simulink model "ex_modeling_signals"  (R2019b)
settings: Solver=VariableStepAuto  StartTime=0.0  StopTime=30  RelTol=1e-3
libraries: simulink x2
settings Model: Creator=The MathWorks, Inc.  LastModifiedBy=The MathWorks, Inc.
settings DataIOCC: ReturnWorkspaceOutputs=off
settings DebuggingCC: PregeneratedLibrarySubsystemCodeDiagnostic=none  ArithmeticOperatorsInVariantConditions=warning
settings SFSimCC: SimUseLocalCustomCode=off  CustomCodeUndefinedFunction=UseInterfaceOnly
settings RTWCC: RTWUseLocalCustomCode=off

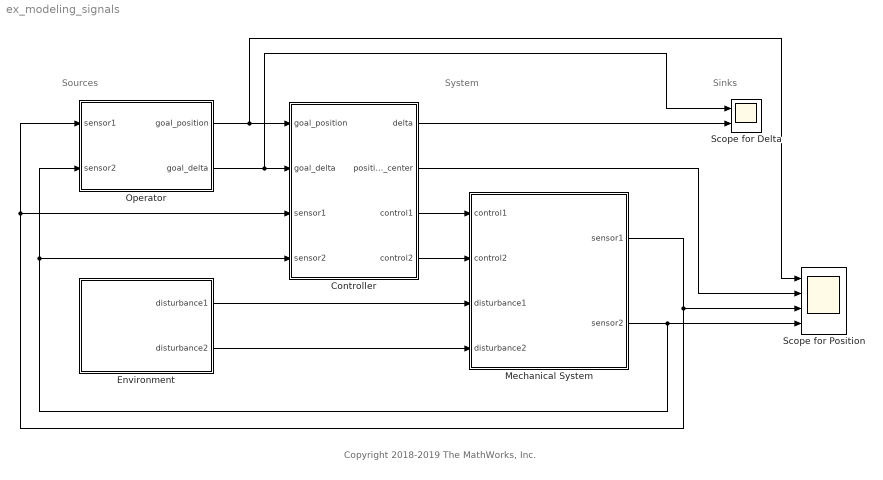
== system ex_modeling_signals ==
  note: System
  note: Sources
  note: Copyright 2018-2019 The MathWorks, Inc.
  note: Sinks
  Controller : Subsystem  TreatAsAtomicUnit=on
  Environment : Subsystem
  Mechanical System : Subsystem
  Operator : Subsystem
  Scope for Delta : Scope  NumInputPorts=2
  Scope for Position : Scope  NumInputPorts=4
  wires:
  Operator/1(goal_position) -> Controller/1(goal_position), Scope for Position/1
  Mechanical System/2(sensor2) -> Operator/2(sensor2), Controller/4(sensor2), Scope for Position/4
  Environment/1(disturbance1) -> Mechanical System/3(disturbance1)
  Environment/2(disturbance2) -> Mechanical System/4(disturbance2)
  Controller/3(control1) -> Mechanical System/1(control1)
  Controller/4(control2) -> Mechanical System/2(control2)
  Controller/2(position_center) -> Scope for Position/2
  Mechanical System/1(sensor1) -> Operator/1(sensor1), Controller/3(sensor1), Scope for Position/3
  Operator/2(goal_delta) -> Controller/2(goal_delta), Scope for Delta/1
  Controller/1(delta) -> Scope for Delta/2

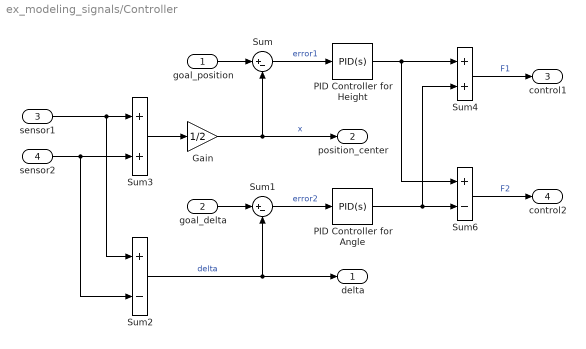
== system ex_modeling_signals/Controller ==
  goal_position : Inport
  goal_delta : Inport  Port=2
  sensor1 : Inport  Port=3
  sensor2 : Inport  Port=4
  Gain : Gain  Gain=1/2
  PID Controller for Angle : simulink/Continuous/PID Controller  Controller=PID  Form=Parallel  TimeDomain=Continuous-time  SampleTime=-1  IntegratorMethod=Forward Euler  FilterMethod=Forward Euler  ControllerParametersSource=internal  P=5.32148000834589  I=3.52799155290048  D=1.99835981321752  UseFilter=on  N=323.232213394405  TunerSelectOption=Transfer Function Based (PID Tuner App)  InitialConditionSource=internal  InitialConditionForIntegrator=0  InitialConditionForFilter=0  DifferentiatorICPrevScaledInput=0  ExternalReset=none  TrackingMode=off  Kt=1  LimitOutput=off  UpperSaturationLimit=inf  LowerSaturationLimit=-inf  LinearizeAsGain=on  AntiWindupMode=none  Kb=1  POutMin=[]  POutMax=[]  IOutMin=[]  IOutMax=[]  DOutMin=[]  DOutMax=[]  NOutMin=[]  NOutMax=[]  SumOutMin=[]  SumOutMax=[]  SaturationOutMin=[]  SaturationOutMax=[]  PParamMin=[]  PParamMax=[]  IParamMin=[]  IParamMax=[]  DParamMin=[]  DParamMax=[]  NParamMin=[]  NParamMax=[]  KbParamMin=[]  KbParamMax=[]  KtParamMin=[]  KtParamMax=[]  KbOutMin=[]  KbOutMax=[]  KtOutMin=[]  KtOutMax=[]  IntegratorOutMin=[]  IntegratorOutMax=[]  FilterOutMin=[]  FilterOutMax=[]  SumI1OutMin=[]  SumI1OutMax=[]  SumI2OutMin=[]  SumI2OutMax=[]  SumI3OutMin=[]  SumI3OutMax=[]  SumI4OutMin=[]  SumI4OutMax=[]  SumDOutMin=[]  SumDOutMax=[]  DifferentiatorOutMin=[]  DifferentiatorOutMax=[]  FilterDiffOutCoefMin=[]  FilterDiffOutCoefMax=[]  ReciprocalOutMin=[]  ReciprocalOutMax=[]  SumDenOutMin=[]  SumDenOutMax=[]  SumNumOutMin=[]  SumNumOutMax=[]  DivideOutMin=[]  DivideOutMax=[]  IntegratorContinuousStateAttributes=''  IntegratorStateMustResolveToSignalObject=off  IntegratorRTWStateStorageClass=Auto  FilterContinuousStateAttributes=''  FilterStateMustResolveToSignalObject=off  FilterRTWStateStorageClass=Auto  ParallelPVariant=InternalParameters  IdealPVariant=Disabled  IVariant=InternalParameters  DVariant=InternalParameters  IntegratorVariant=Continuous  SatVariant=Disabled  AWVariant=Passthrough  PCopyVariant=Disabled  TRVariant=Disabled  FdbkBlocksVariant=Forward  IdealPFdbkVariant=Disabled  SatFdbkVariant=Disabled  DerivativeFilterVariant=ContFilter  NVariant=InternalParameters  NCopyVariant=Disabled  FilterICVariant=InternalICsFilter  IntegratorICVariant=InternalICs  ExternalResetVariant=Disabled  TRSumVariant=Passthrough  SumFdbkVariant=Disabled  SumVariant=Sum_PID
  PID Controller for Height : simulink/Continuous/PID Controller  Controller=PID  Form=Parallel  TimeDomain=Continuous-time  SampleTime=-1  IntegratorMethod=Forward Euler  FilterMethod=Forward Euler  ControllerParametersSource=internal  P=23.792676457344  I=17.7497318502065  D=7.56800739635058  UseFilter=on  N=49.2376691493838  TunerSelectOption=Transfer Function Based (PID Tuner App)  InitialConditionSource=internal  InitialConditionForIntegrator=0  InitialConditionForFilter=0  DifferentiatorICPrevScaledInput=0  ExternalReset=none  TrackingMode=off  Kt=1  LimitOutput=off  UpperSaturationLimit=inf  LowerSaturationLimit=-inf  LinearizeAsGain=on  AntiWindupMode=none  Kb=1  POutMin=[]  POutMax=[]  IOutMin=[]  IOutMax=[]  DOutMin=[]  DOutMax=[]  NOutMin=[]  NOutMax=[]  SumOutMin=[]  SumOutMax=[]  SaturationOutMin=[]  SaturationOutMax=[]  PParamMin=[]  PParamMax=[]  IParamMin=[]  IParamMax=[]  DParamMin=[]  DParamMax=[]  NParamMin=[]  NParamMax=[]  KbParamMin=[]  KbParamMax=[]  KtParamMin=[]  KtParamMax=[]  KbOutMin=[]  KbOutMax=[]  KtOutMin=[]  KtOutMax=[]  IntegratorOutMin=[]  IntegratorOutMax=[]  FilterOutMin=[]  FilterOutMax=[]  SumI1OutMin=[]  SumI1OutMax=[]  SumI2OutMin=[]  SumI2OutMax=[]  SumI3OutMin=[]  SumI3OutMax=[]  SumI4OutMin=[]  SumI4OutMax=[]  SumDOutMin=[]  SumDOutMax=[]  DifferentiatorOutMin=[]  DifferentiatorOutMax=[]  FilterDiffOutCoefMin=[]  FilterDiffOutCoefMax=[]  ReciprocalOutMin=[]  ReciprocalOutMax=[]  SumDenOutMin=[]  SumDenOutMax=[]  SumNumOutMin=[]  SumNumOutMax=[]  DivideOutMin=[]  DivideOutMax=[]  IntegratorContinuousStateAttributes=''  IntegratorStateMustResolveToSignalObject=off  IntegratorRTWStateStorageClass=Auto  FilterContinuousStateAttributes=''  FilterStateMustResolveToSignalObject=off  FilterRTWStateStorageClass=Auto  ParallelPVariant=InternalParameters  IdealPVariant=Disabled  IVariant=InternalParameters  DVariant=InternalParameters  IntegratorVariant=Continuous  SatVariant=Disabled  AWVariant=Passthrough  PCopyVariant=Disabled  TRVariant=Disabled  FdbkBlocksVariant=Forward  IdealPFdbkVariant=Disabled  SatFdbkVariant=Disabled  DerivativeFilterVariant=ContFilter  NVariant=InternalParameters  NCopyVariant=Disabled  FilterICVariant=InternalICsFilter  IntegratorICVariant=InternalICs  ExternalResetVariant=Disabled  TRSumVariant=Passthrough  SumFdbkVariant=Disabled  SumVariant=Sum_PID
  Sum : Sum  Inputs=|+-
  Sum1 : Sum  Inputs=|+-
  Sum2 : Sum  Inputs=+-
  Sum3 : Sum
  Sum4 : Sum
  Sum6 : Sum  Inputs=+-
  delta : Outport  VectorParamsAs1DForOutWhenUnconnected=off
  position_center : Outport  Port=2  VectorParamsAs1DForOutWhenUnconnected=off
  control1 : Outport  Port=3  VectorParamsAs1DForOutWhenUnconnected=off
  control2 : Outport  Port=4  VectorParamsAs1DForOutWhenUnconnected=off
  wires:
  PID Controller for Height/1 -> Sum6/1, Sum4/1
  Sum6/1 -> control2/1  "F2"
  Sum/1 -> PID Controller for Height/1  "error1"
  goal_delta/1 -> Sum1/1
  PID Controller for Angle/1 -> Sum6/2, Sum4/2
  Sum1/1 -> PID Controller for Angle/1  "error2"
  Sum4/1 -> control1/1  "F1"
  goal_position/1 -> Sum/1
  Sum2/1 -> delta/1, Sum1/2  "delta"
  sensor1/1 -> Sum2/1, Sum3/1
  sensor2/1 -> Sum2/2, Sum3/2
  Gain/1 -> position_center/1, Sum/2  "x"
  Sum3/1 -> Gain/1

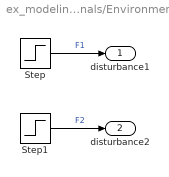
== system ex_modeling_signals/Environment ==
  Step : Step  Time=10  After=10  SampleTime=0
  Step1 : Step  Time=20  After=10  SampleTime=0
  disturbance1 : Outport  VectorParamsAs1DForOutWhenUnconnected=off
  disturbance2 : Outport  Port=2  VectorParamsAs1DForOutWhenUnconnected=off
  wires:
  Step/1 -> disturbance1/1  "F1"
  Step1/1 -> disturbance2/1  "F2"

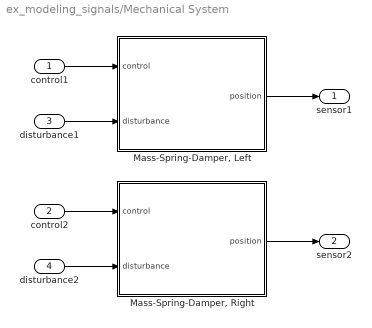
== system ex_modeling_signals/Mechanical System ==
  control1 : Inport
  control2 : Inport  Port=2
  disturbance1 : Inport  Port=3
  disturbance2 : Inport  Port=4
  "Mass-Spring-Damper, Left" : Subsystem
  "Mass-Spring-Damper, Right" : Subsystem
  sensor1 : Outport  VectorParamsAs1DForOutWhenUnconnected=off
  sensor2 : Outport  Port=2  VectorParamsAs1DForOutWhenUnconnected=off
  wires:
  control1/1 -> "Mass-Spring-Damper, Left"/1(control)
  control2/1 -> "Mass-Spring-Damper, Right"/1(control)
  disturbance1/1 -> "Mass-Spring-Damper, Left"/2(disturbance)
  disturbance2/1 -> "Mass-Spring-Damper, Right"/2(disturbance)
  "Mass-Spring-Damper, Left"/1(position) -> sensor1/1
  "Mass-Spring-Damper, Right"/1(position) -> sensor2/1

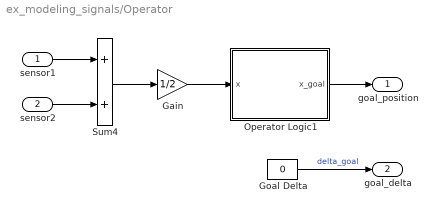
== system ex_modeling_signals/Operator ==
  sensor1 : Inport
  sensor2 : Inport  Port=2
  Gain : Gain  Gain=1/2
  Goal Delta : Constant  Value=0
  Operator Logic1 : Stateflow chart  TreatAsAtomicUnit=on
  Sum4 : Sum
  goal_position : Outport  VectorParamsAs1DForOutWhenUnconnected=off
  goal_delta : Outport  Port=2  VectorParamsAs1DForOutWhenUnconnected=off
  wires:
  Operator Logic1/1(x_goal) -> goal_position/1
  Sum4/1 -> Gain/1
  Gain/1 -> Operator Logic1/1(x)
  sensor2/1 -> Sum4/2
  sensor1/1 -> Sum4/1
  Goal Delta/1 -> goal_delta/1  "delta_goal"

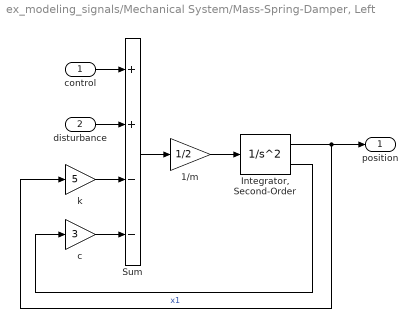
== system ex_modeling_signals/Mechanical System/Mass-Spring-Damper, Left ==
  control : Inport
  disturbance : Inport  Port=2
  1/m : Gain  Gain=1/2
  "Integrator, Second-Order" : SecondOrderIntegrator
  Sum : Sum  Inputs=++--
  c : Gain  Gain=3
  k : Gain  Gain=5
  position : Outport  VectorParamsAs1DForOutWhenUnconnected=off
  wires:
  k/1 -> Sum/3
  control/1 -> Sum/1
  "Integrator, Second-Order"/1 -> position/1, k/1  "x1"
  c/1 -> Sum/4
  "Integrator, Second-Order"/2 -> c/1
  disturbance/1 -> Sum/2
  1/m/1 -> "Integrator, Second-Order"/1
  Sum/1 -> 1/m/1

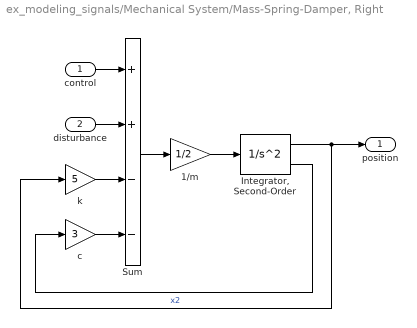
== system ex_modeling_signals/Mechanical System/Mass-Spring-Damper, Right ==
  control : Inport
  disturbance : Inport  Port=2
  1/m : Gain  Gain=1/2
  "Integrator, Second-Order" : SecondOrderIntegrator
  Sum : Sum  Inputs=++--
  c : Gain  Gain=3
  k : Gain  Gain=5
  position : Outport  VectorParamsAs1DForOutWhenUnconnected=off
  wires:
  Sum/1 -> 1/m/1
  1/m/1 -> "Integrator, Second-Order"/1
  disturbance/1 -> Sum/2
  "Integrator, Second-Order"/2 -> c/1
  c/1 -> Sum/4
  "Integrator, Second-Order"/1 -> k/1, position/1  "x2"
  control/1 -> Sum/1
  k/1 -> Sum/3

== stateflow chart ex_modeling_signals/Operator/Operator Logic1 ==
  state wait
    entry: x_goal = 0;
  state FirstOperation
    entry: x_goal = 2;
  state SecondOperation
    entry: x_goal = 1;
  wait -> FirstOperation : after(2,sec)
  FirstOperation -> SecondOperation : [x>2]
  (default) -> wait
  data: x input; x_goal output
